simulink model "q_sip_swingup"  (Simulink 7.9)
settings: Solver=ode1  StartTime=0.0  StopTime=inf  FixedStep=0.002  RelTol=1e-3
values from neighbouring files (symbols this model uses):
  epsilon = 10.0 * pi / 180    (= 0.174532925199)    [setup_ip02_sip.m]
  Er = 2*Mp*lp*9.81    [d_swing_up.m]
  g = 9.81    [config_sp.m]
  Jp = Mp * Lp^2 / 12    [config_sp.m]
  K_AMP = 1    [setup_ip02_sip.m]
  lp = 7 * K_IN2M    [config_sp.m]
  Mp = 0.127    [config_sp.m]
  VMAX_DAC = 10    [setup_ip02_sip.m]
  wcf = 2 * pi * 10.0    (= 62.8318530718)    [setup_ip02_sip.m]
  X_LIM_ENABLE = 1    [setup_ip02_sip.m]
  X_MAX = 0.3    [setup_ip02_sip.m]
  X_MIN = - X_MAX    (= -0.3)    [setup_ip02_sip.m]
  zetaf = 0.9    [setup_ip02_sip.m]
undefined symbols (not defined in the file or in its folder): eta_g, eta_m, HIL, K, K_EC, K_EP, Kg, Km, Kt, Mc, qc_get_step_size, r_mp, Rm, VMAX_AMP
libraries: quarc_library x6, simulink x3, simulink_extras x2
settings Model: Creator=MLevis  LastModifiedBy=mkrug  SimulationMode=external  ExtModeTrigDuration=10000  BufferReuse=off
settings SolverCC: PositivePriorityOrder=on
settings OptimizationCC: BooleanDataType=off  InlineInvariantSignals=on  OptimizeBlockIOStorage=off  BufferReuse=off  ExpressionFolding=off  LocalBlockOutputs=off  InitFltsAndDblsToZero=on
settings DebuggingCC: SaveWithParameterizedLinksMsg=none  SignalResolutionControl=TryResolveAllWithWarning  SolverPrmCheckMsg=none  MultiTaskDSMMsg=warning  MultiTaskCondExecSysMsg=none  FcnCallInpInsideContextMsg=Use local settings  StrictBusMsg=None
settings HardwareCC: TargetHWDeviceType=32-bit Generic
settings SFSimCC: SimParseCustomCode=off
settings RTWCC: SystemTargetFile=quarc_windows.tlc  TemplateMakefile=quarc_default_tmf  Description=Quarc Win32 Target  ProcessScript=quarc_windows_make_rtw_hook  IncludeERTFirstTime=on
settings STFCustomTargetCC: TargetFcnLib=ansi_tfl_tmw.mat  TargetPreCompLibLocation=C:\PROGRA~3\QUARC\lib\2012a\windows\release  CodeReplacementLibrary=ANSI_C  GeneratePreprocessorConditionals=Disable all  SystemTargetFile=quarc_windows.tlc
settings GRTTargetCC: TargetFcnLib=ansi_tfl_tmw.mat  TargetPreCompLibLocation=C:\PROGRA~3\QUARC\lib\2012a\windows\release  ParMdlRefBuildCompliant=off  CompOptLevelCompliant=off  ConcurrentExecutionCompliant=off  CombineOutputUpdateFcns=off  MatFileLogging=off  GRTInterface=on  ExtMode=on  ExtModeMexFile=quarc_comm

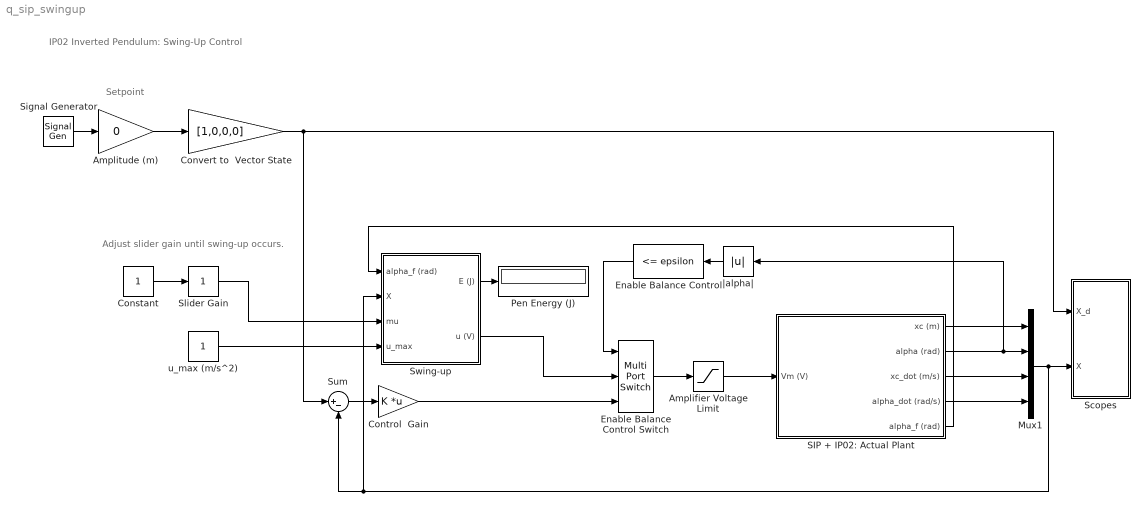
== system q_sip_swingup ==
  note: Setpoint
  note: IP02 Inverted Pendulum: Swing-Up Control
  note: Adjust slider gain
      | until swing-up occurs.
  Amplifier Voltage Limit : Saturate  UpperLimit=VMAX_AMP  LowerLimit=- VMAX_AMP
  Amplitude (m) : Gain  Gain=0  SaturateOnIntegerOverflow=on  OutDataTypeStr=Inherit: Same as input  ParamDataTypeStr=Inherit: Same as input
  Constant : Constant
  Control  Gain : Gain  Gain=K  Multiplication=Matrix(K*u)
  Convert to  Vector State : Gain  Gain=[1,0,0,0]
  Enable Balance Control : simulink/Logic and Bit Operations/Compare To Constant  relop=<=  const=epsilon  OutDataTypeStr=uint8  ZeroCross=off
  Enable Balance Control Switch : MultiPortSwitch  DataPortOrder=Zero-based contiguous  Inputs=2  zeroidx=on
  Mux1 : Mux
  Pen Energy (J) : Display
      settings: Decimation=100
  SIP + IP02: Actual Plant : Subsystem
  Scopes : Subsystem
  Signal Generator : SignalGenerator  WaveForm=square  Frequency=0.1
  Slider Gain : simulink/Math Operations/Slider Gain  low=0  gain=1  high=20
  Sum : Sum  Inputs=|+-
  Swing-up : Subsystem
  u_max (m/s^2) : Constant
  |alpha| : Abs
  wires:
  Amplitude (m)/1 -> Convert to  Vector State/1
  Signal Generator/1 -> Amplitude (m)/1
  Convert to  Vector State/1 -> Scopes/1(X_d), Sum/1
  Sum/1 -> Control  Gain/1
  Enable Balance Control Switch/1 -> Amplifier Voltage Limit/1
  Control  Gain/1 -> Enable Balance Control Switch/3
  |alpha|/1 -> Enable Balance Control/1
  Enable Balance Control/1 -> Enable Balance Control Switch/1
  Constant/1 -> Slider Gain/1
  Slider Gain/1 -> Swing-up/3(mu)
  Swing-up/1(E (J)) -> Pen Energy (J)/1
  u_max (m/s^2)/1 -> Swing-up/4(u_max)
  Amplifier Voltage Limit/1 -> SIP + IP02: Actual Plant/1(Vm (V))
  SIP + IP02: Actual Plant/1(xc (m)) -> Mux1/1
  SIP + IP02: Actual Plant/2(alpha (rad)) -> Mux1/2, |alpha|/1
  SIP + IP02: Actual Plant/3(xc_dot (m/s)) -> Mux1/3
  SIP + IP02: Actual Plant/4(alpha_dot (rad/s)) -> Mux1/4
  Mux1/1 -> Scopes/2(X), Sum/2, Swing-up/2(X)
  SIP + IP02: Actual Plant/5(alpha_f (rad)) -> Swing-up/1(alpha_f (rad))
  Swing-up/2(u (V)) -> Enable Balance Control Switch/2

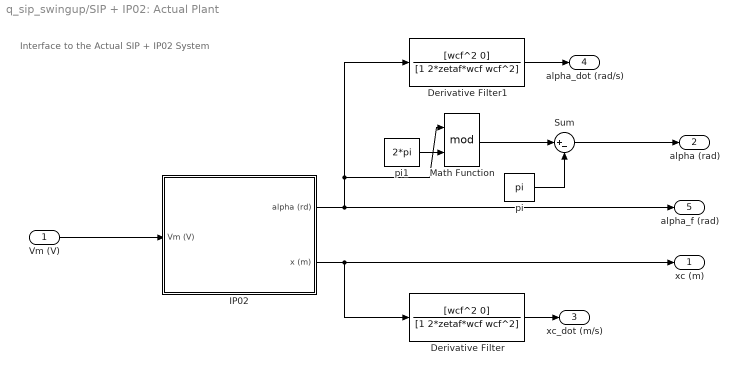
== system q_sip_swingup/SIP + IP02: Actual Plant ==
  note: Interface to the Actual
      | SIP + IP02 System
  Vm (V) : Inport
  Derivative Filter : TransferFcn  Numerator=[wcf^2 0]  Denominator=[1 2*zetaf*wcf wcf^2]
  Derivative Filter1 : TransferFcn  Numerator=[wcf^2 0]  Denominator=[1 2*zetaf*wcf wcf^2]
  "IP02 " : Subsystem
  Math Function : Math  Operator=mod  SaturateOnIntegerOverflow=on
  Sum : Sum  Inputs=|+-  SaturateOnIntegerOverflow=on  InputSameDT=on  OutDataTypeStr=Inherit: Same as first input
  pi : Constant  Value=pi
  pi1 : Constant  Value=2*pi
  xc (m) : Outport  InitialOutput=0
  alpha (rad) : Outport  Port=2  InitialOutput=0
  xc_dot (m/s) : Outport  Port=3  InitialOutput=0
  alpha_dot (rad/s) : Outport  Port=4  InitialOutput=0
  alpha_f (rad) : Outport  Port=5  InitialOutput=0
  wires:
  "IP02 "/2(x (m)) -> xc (m)/1, Derivative Filter/1
  Derivative Filter1/1 -> alpha_dot (rad/s)/1
  "IP02 "/1(alpha (rd)) -> Derivative Filter1/1, Math Function/1, alpha_f (rad)/1
  Derivative Filter/1 -> xc_dot (m/s)/1
  pi1/1 -> Math Function/2
  pi/1 -> Sum/2
  Sum/1 -> alpha (rad)/1
  Math Function/1 -> Sum/1
  Vm (V)/1 -> "IP02 "/1(Vm (V))

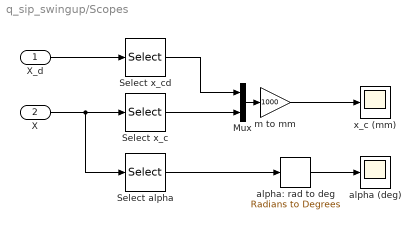
== system q_sip_swingup/Scopes ==
  X_d : Inport
  X : Inport  Port=2
  Mux : Mux  Inputs=2
  Select alpha : Selector  InputPortWidth=4  IndexOptions=Index vector (dialog)  Indices=2  OutputSizes=[(-2)]
  Select x_c : Selector  InputPortWidth=4  IndexOptions=Index vector (dialog)  Indices=1  OutputSizes=[(-2)]
  Select x_cd : Selector  InputPortWidth=4  IndexOptions=Index vector (dialog)  Indices=1  OutputSizes=[(-2)]
  alpha (deg) : Scope
      settings: TimeRange=20  YMin=-200  YMax=200  SaveName=data_alpha  MaxDataPoints=20000
  alpha: rad to deg : simulink_extras/Transformations/Radians to Degrees
  m to mm : Gain  Gain=1000
  x_c (mm) : Scope
      settings: TimeRange=20  YMin=-0  YMax=13  SaveName=data_xc  MaxDataPoints=20000
  wires:
  X_d/1 -> Select x_cd/1
  Select alpha/1 -> alpha: rad to deg/1
  alpha: rad to deg/1 -> alpha (deg)/1
  X/1 -> Select alpha/1, Select x_c/1
  Select x_cd/1 -> Mux/1
  m to mm/1 -> x_c (mm)/1
  Select x_c/1 -> Mux/2
  Mux/1 -> m to mm/1

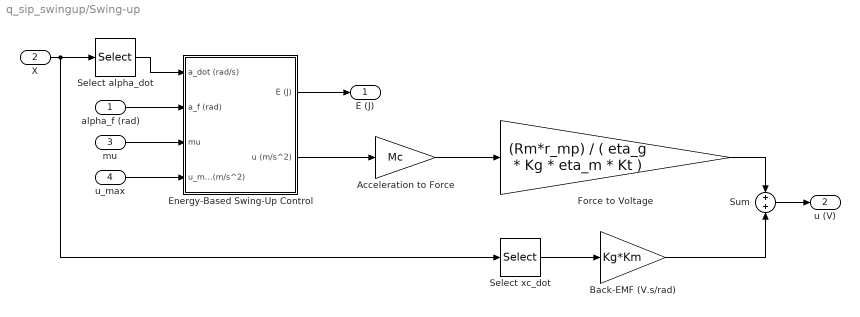
== system q_sip_swingup/Swing-up ==
  alpha_f (rad) : Inport
  X : Inport  Port=2
  mu : Inport  Port=3
  u_max : Inport  Port=4
  Acceleration to Force : Gain  Gain=Mc
  Back-EMF (V.s/rad) : Gain  Gain=Kg*Km
  Energy-Based Swing-Up Control : Subsystem
  Force to Voltage : Gain  Gain=(Rm*r_mp) / ( eta_g * Kg * eta_m * Kt )
  Select alpha_dot : Selector  InputPortWidth=4  IndexOptions=Index vector (dialog)  Indices=[4]  OutputSizes=1
  Select xc_dot : Selector  InputPortWidth=4  IndexOptions=Index vector (dialog)  Indices=[3]  OutputSizes=1
  Sum : Sum
  E (J) : Outport
  u (V) : Outport  Port=2
  wires:
  Energy-Based Swing-Up Control/2(u (m/s^2)) -> Acceleration to Force/1
  Acceleration to Force/1 -> Force to Voltage/1
  Energy-Based Swing-Up Control/1(E (J)) -> E (J)/1
  alpha_f (rad)/1 -> Energy-Based Swing-Up Control/2(a_f (rad))
  mu/1 -> Energy-Based Swing-Up Control/3(mu)
  Select alpha_dot/1 -> Energy-Based Swing-Up Control/1(a_dot (rad/s))
  X/1 -> Select alpha_dot/1, Select xc_dot/1
  u_max/1 -> Energy-Based Swing-Up Control/4(u_max (m/s^2))
  Select xc_dot/1 -> Back-EMF (V.s/rad)/1
  Force to Voltage/1 -> Sum/1
  Back-EMF (V.s/rad)/1 -> Sum/2
  Sum/1 -> u (V)/1

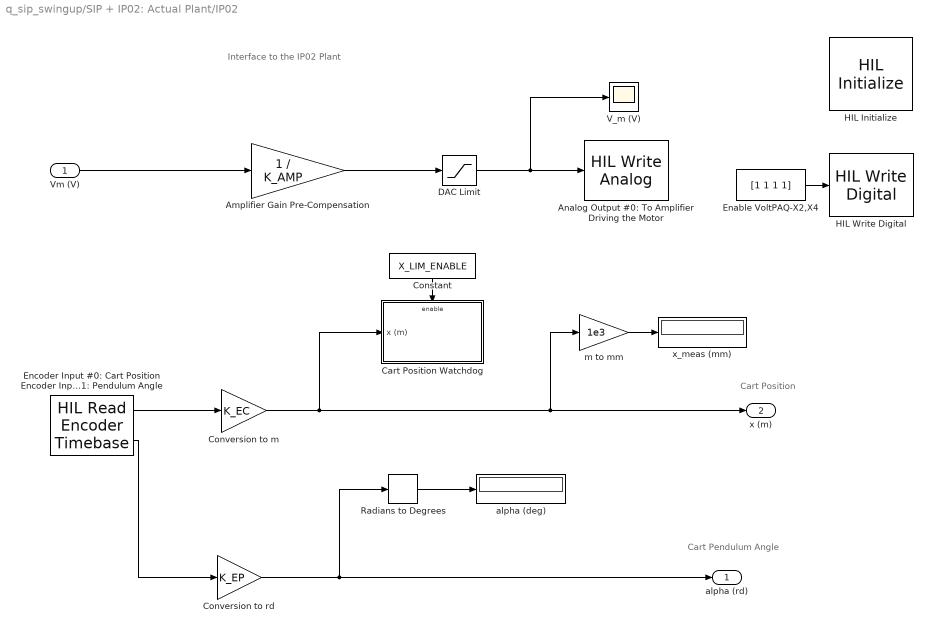
== system q_sip_swingup/SIP + IP02: Actual Plant/IP02  ==
  note: Cart Pendulum Angle
  note: Cart Position
  note: Interface to the IP02 Plant
  Vm (V) : Inport
  Amplifier Gain Pre-Compensation : Gain  Gain=1 / K_AMP  SaturateOnIntegerOverflow=on  OutDataTypeStr=Inherit: Same as input  ParamDataTypeStr=Inherit: Same as input
  Analog Output #0: To Amplifier Driving the Motor : quarc_library/Data Acquisition/Generic/Immediate I//O/HIL Write Analog  Tag=unassigned  object_name=HIL-1  channels=0  sample_time=-1  active=on  vector_input=on
  Cart Position Watchdog : Subsystem  TreatAsAtomicUnit=on
  Constant : Constant  Value=X_LIM_ENABLE
  Conversion to m : Gain  Gain=K_EC  SaturateOnIntegerOverflow=on  OutDataTypeStr=Inherit: Same as input  ParamDataTypeStr=Inherit: Same as input
  Conversion to rd : Gain  Gain=K_EP  SaturateOnIntegerOverflow=on  OutDataTypeStr=Inherit: Same as input  ParamDataTypeStr=Inherit: Same as input
  DAC Limit : Saturate  UpperLimit=VMAX_DAC  LowerLimit=- VMAX_DAC
  Enable VoltPAQ-X2,X4 : Constant  Value=[1 1 1 1]
  Encoder Input #0: Cart Position Encoder Input #1: Pendulum Angle : quarc_library/Data Acquisition/Generic/Timebases/HIL Read Encoder Timebase  Tag=unassigned  object_name=HIL-1  clock=0  channels=[0 1]  samples_in_buffer=max(ceil(1/qc_get_step_size), 1)  active=on  vector_output=off  data_type_mode=Inherit via back propagation  data_type=double
  HIL Initialize : quarc_library/Data Acquisition/Generic/Configuration/HIL Initialize  object_name=HIL-1  board_type=q2_usb  board_number=0  board_options=d0=digital;d1=digital;led=auto;update_rate=normal  exclusive=off  active=off  hardware_clocks=[0:2]  clock_modes=[]  initial_clock_frequencies=[]  set_clock_params_at_start=off  set_clock_params_at_switch_in=off  set_clock_frequencies_at_start=off  set_clock_frequencies_at_switch_in=off  analog_input_channels=[0:1]  analog_input_maximums=10  analog_input_minimums=-10  set_analog_input_params_at_start=on  set_analog_input_params_at_switch_in=off  analog_output_channels=[0:1]  analog_output_maximums=10  analog_output_minimums=-10  initial_analog_outputs=[0]  final_analog_outputs=[0]  watchdog_analog_outputs=0  set_analog_output_params_at_start=on  set_analog_output_params_at_switch_in=off  set_analog_outputs_at_start=on  set_analog_outputs_at_switch_in=off  set_analog_outputs_at_terminate=on  set_analog_outputs_at_switch_out=off  set_analog_outputs_on_watchdog=off  digital_input_channels=[]  digital_output_channels=[0:7]  digital_output_configuration=[]  initial_digital_outputs=[0]  final_digital_outputs=[0]  watchdog_digital_outputs=[0]  set_digital_output_params_at_start=off  set_digital_output_params_at_switch_in=off  set_digital_outputs_at_start=on  set_digital_outputs_at_switch_in=off  set_digital_outputs_at_terminate=on  set_digital_outputs_at_switch_out=off  set_digital_outputs_on_watchdog=off  encoder_channels=[0:1]  quadrature=[4]  encoder_filter_frequency=[]  initial_encoder_counts=[0]  set_encoder_params_at_start=on  set_encoder_params_at_switch_in=off  set_encoder_counts_at_start=on  set_encoder_counts_at_switch_in=off  pwm_channels=[]  pwm_modes=[0]  pwm_frequency=1/0.020  pwm_configuration=[]  pwm_alignment=[]  pwm_polarity=[]  pwm_leading_deadband=[]  pwm_trailing_deadband=[]  initial_pwm_outputs=[0]  final_pwm_outputs=[0]  watchdog_pwm_outputs=[0]  set_pwm_params_at_start=on  set_pwm_params_at_switch_in=off  set_pwm_outputs_at_start=on  set_pwm_outputs_at_switch_in=off  set_pwm_outputs_at_terminate=on  set_pwm_outputs_at_switch_out=off  set_pwm_outputs_on_watchdog=off  other_output_channels=[]  initial_other_outputs=[]  final_other_outputs=[]  watchdog_other_outputs=[]  set_other_outputs_at_start=off  set_other_outputs_at_switch_in=off  set_other_outputs_at_terminate=off  set_other_outputs_at_switch_out=off  set_other_outputs_on_watchdog=off
  HIL Write Digital : quarc_library/Data Acquisition/Generic/Immediate I//O/HIL Write Digital  object_name=HIL-1  channels=[0:3]  sample_time=-1  active=off  vector_input=on
  Radians to Degrees : simulink_extras/Transformations/Radians to Degrees
  V_m (V) : Scope
      settings: TickLabels=on  TimeRange=20  YMin=-550000  YMax=50000  SaveName=data_Vm  MaxDataPoints=20000
  alpha (deg) : Display
      settings: Decimation=100
  m to mm : Gain  Gain=1e3  SaturateOnIntegerOverflow=on  OutDataTypeStr=Inherit: Same as input  ParamDataTypeStr=Inherit: Same as input
  x_meas (mm) : Display
      settings: Decimation=100
  alpha (rd) : Outport  InitialOutput=0
  x (m) : Outport  Port=2  InitialOutput=0
  wires:
  Encoder Input #0: Cart Position Encoder Input #1: Pendulum Angle/1 -> Conversion to m/1
  Conversion to m/1 -> Cart Position Watchdog/1(x (m)), x (m)/1, m to mm/1
  Amplifier Gain Pre-Compensation/1 -> DAC Limit/1
  m to mm/1 -> x_meas (mm)/1
  Encoder Input #0: Cart Position Encoder Input #1: Pendulum Angle/2 -> Conversion to rd/1
  Radians to Degrees/1 -> alpha (deg)/1
  Conversion to rd/1 -> Radians to Degrees/1, alpha (rd)/1
  Constant/1 -> Cart Position Watchdog/Enable
  DAC Limit/1 -> Analog Output #0: To Amplifier Driving the Motor/1, V_m (V)/1
  Vm (V)/1 -> Amplifier Gain Pre-Compensation/1
  Enable VoltPAQ-X2,X4/1 -> HIL Write Digital/1

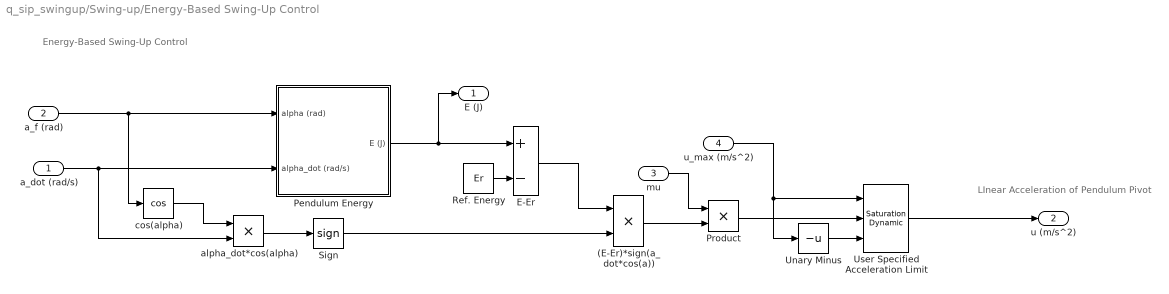
== system q_sip_swingup/Swing-up/Energy-Based Swing-Up Control ==
  note: Energy-Based Swing-Up Control
  note: LInear Acceleration of
      | Pendulum Pivot
  a_dot (rad/s) : Inport
  a_f (rad) : Inport  Port=2
  mu : Inport  Port=3
  u_max (m/s^2) : Inport  Port=4
  (E-Er)*sign(a_dot*cos(a)) : Product  RndMeth=Zero
  E-Er : Sum  Inputs=+-
  Pendulum Energy : Subsystem
  Product : Product  RndMeth=Zero
  Ref. Energy : Constant  Value=Er
  Sign : Signum
  Unary Minus : UnaryMinus
  User Specified Acceleration Limit : simulink/Discontinuities/Saturation Dynamic  OutMin=[]  OutMax=[]  OutDataTypeStr=Inherit: Same as second input  OutDataType=fixdt(1, 16)  OutScaling=2^-10  DoSatur=off
  alpha_dot*cos(alpha) : Product  RndMeth=Zero
  cos(alpha) : Trigonometry  Operator=cos
  E (J) : Outport
  u (m/s^2) : Outport  Port=2
  wires:
  alpha_dot*cos(alpha)/1 -> Sign/1
  Sign/1 -> (E-Er)*sign(a_dot*cos(a))/2
  cos(alpha)/1 -> alpha_dot*cos(alpha)/1
  a_f (rad)/1 -> cos(alpha)/1, Pendulum Energy/1(alpha (rad))
  E-Er/1 -> (E-Er)*sign(a_dot*cos(a))/1
  Pendulum Energy/1(E (J)) -> E (J)/1, E-Er/1
  a_dot (rad/s)/1 -> alpha_dot*cos(alpha)/2, Pendulum Energy/2(alpha_dot (rad/s))
  (E-Er)*sign(a_dot*cos(a))/1 -> Product/2
  Ref. Energy/1 -> E-Er/2
  mu/1 -> Product/1
  Product/1 -> User Specified Acceleration Limit/2
  u_max (m/s^2)/1 -> User Specified Acceleration Limit/1, Unary Minus/1
  Unary Minus/1 -> User Specified Acceleration Limit/3
  User Specified Acceleration Limit/1 -> u (m/s^2)/1

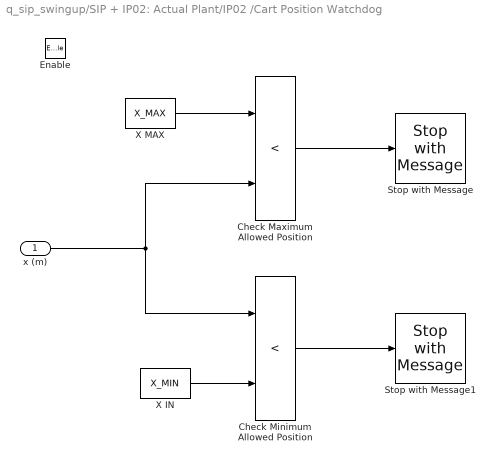
== system q_sip_swingup/SIP + IP02: Actual Plant/IP02 /Cart Position Watchdog ==
  x (m) : Inport
  Enable : EnablePort
  Check Maximum Allowed Position : RelationalOperator  Operator=<  InputSameDT=on
  Check Minimum Allowed Position : RelationalOperator  Operator=<  InputSameDT=on
  Stop with Message : quarc_library/Sinks/Error Handling/Stop with Message  message_type=Fixed error message  message_icon=Error  message=Maximum Limit Reached.
  Stop with Message1 : quarc_library/Sinks/Error Handling/Stop with Message  message_type=Fixed error message  message_icon=Error  message=Minimum Limit Reached.
  X IN : Constant  Value=X_MIN
  X MAX : Constant  Value=X_MAX
  wires:
  Check Maximum Allowed Position/1 -> Stop with Message/1
  x (m)/1 -> Check Minimum Allowed Position/1, Check Maximum Allowed Position/2
  X IN/1 -> Check Minimum Allowed Position/2
  Check Minimum Allowed Position/1 -> Stop with Message1/1
  X MAX/1 -> Check Maximum Allowed Position/1

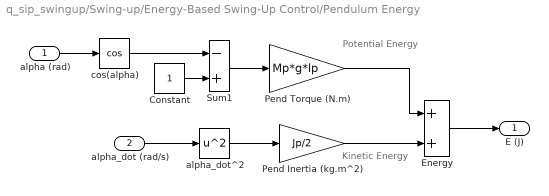
== system q_sip_swingup/Swing-up/Energy-Based Swing-Up Control/Pendulum Energy ==
  note: Kinetic Energy
  note: Potential Energy
  alpha (rad) : Inport
  alpha_dot (rad/s) : Inport  Port=2
  Constant : Constant
  Energy : Sum  SaturateOnIntegerOverflow=on
  Pend Inertia (kg.m^2) : Gain  Gain=Jp/2
  Pend Torque (N.m) : Gain  Gain=Mp*g*lp
  Sum1 : Sum  Inputs=-+  SaturateOnIntegerOverflow=on
  alpha_dot^2 : Math  Operator=square  SaturateOnIntegerOverflow=on
  cos(alpha) : Trigonometry  Operator=cos
  E (J) : Outport
  wires:
  Constant/1 -> Sum1/2
  Pend Inertia (kg.m^2)/1 -> Energy/2
  Sum1/1 -> Pend Torque (N.m)/1
  alpha_dot^2/1 -> Pend Inertia (kg.m^2)/1
  Pend Torque (N.m)/1 -> Energy/1
  alpha (rad)/1 -> cos(alpha)/1
  alpha_dot (rad/s)/1 -> alpha_dot^2/1
  Energy/1 -> E (J)/1
  cos(alpha)/1 -> Sum1/1
